simulink model "AirSpringModel"  (R2025a)
settings: Solver=VariableStepAuto  StartTime=0.0  StopTime=10  MaxStep=0.003  MinStep=0.001  RelTol=1e-3
values from neighbouring files (symbols this model uses):
  c = 1200    [Air_pressure.m]
  m = 300    [Air_pressure.m]
settings Model: Creator=omrez  LastModifiedBy=omrez

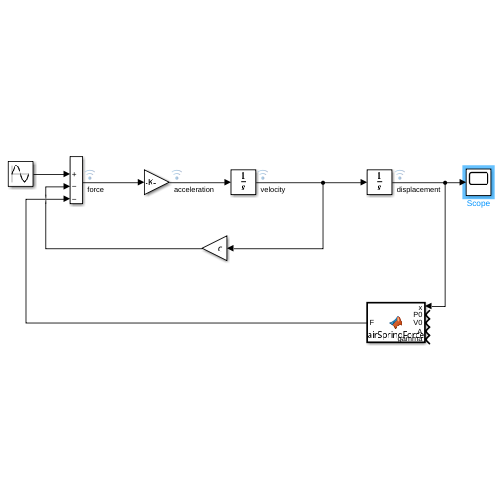
[thumbnail: Simulink's stored preview of the top-level diagram]
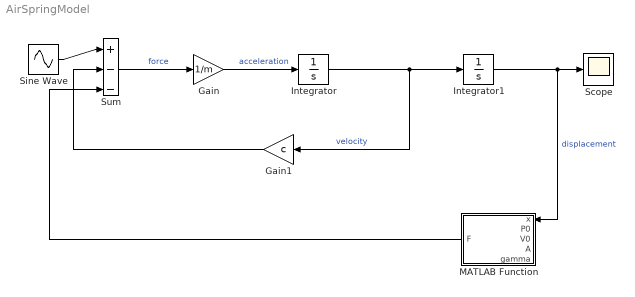
== system AirSpringModel ==
  Gain : Gain  Gain=1/m
  Gain1 : Gain  Gain=c
  Integrator : Integrator
  Integrator1 : Integrator
  MATLAB Function : MATLAB Function  TreatAsAtomicUnit=on
  Scope : Scope
      settings: ActiveDisplayYMinimum=-1  ActiveDisplayYMaximum=1
  Sine Wave : Sin  Amplitude=10  Frequency=10  SampleTime=0
  Sum : Sum  Inputs=|+--
  wires:
  Gain/1 -> Integrator/1  "acceleration"
  Sum/1 -> Gain/1  "force"
  Sine Wave/1 -> Sum/1
  Integrator/1 -> Gain1/1, Integrator1/1  "velocity"
  Integrator1/1 -> MATLAB Function/1(x), Scope/1  "displacement"
  MATLAB Function/1(F) -> Sum/3
  Gain1/1 -> Sum/2

== matlab function AirSpringModel/MATLAB Function ==
  data: x input; F output; P0 input; V0 input; A input; gamma input
function F = airSpringForce(x, P0, V0, A, gamma)
% Nonlinear Air Spring Force Model
% x = displacement
% P0 = initial pressure
% V0 = initial chamber volume
% A = diaphragm area
% gamma = polytropic index


    % Avoid division by zero
    if V0 - A*x <= 0
        F = 0;  % or a very small value
    else
        F = (gamma*P0*A^2)/(V0 - A*x) * x;
    end
end
